simulink model "gm_sampleModel1995_3_sub_sub"  (R2023a)
settings: Solver=VariableStepAuto  StartTime=0.0  StopTime=10.0  RelTol=1e-3
libraries: hdlsllib x3, simulink x1
settings Model: Creator=user1  LastModifiedBy=user1
settings OptimizationCC: BlockReduction=off  ConditionallyExecuteInputs=off
settings DebuggingCC: InheritedTsInSrcMsg=none

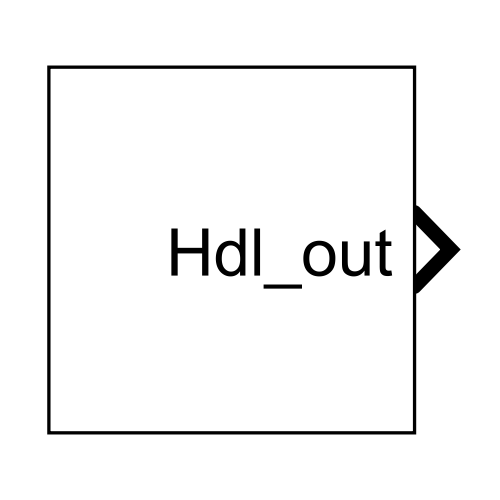
[thumbnail: Simulink's stored preview of the top-level diagram]
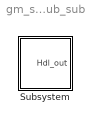
== system gm_sampleModel1995_3_sub_sub ==
  Subsystem : Subsystem

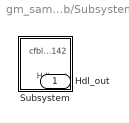
== system gm_sampleModel1995_3_sub_sub/Subsystem ==
  Subsystem : Subsystem
  Hdl_out : Outport  OutDataTypeStr=uint8

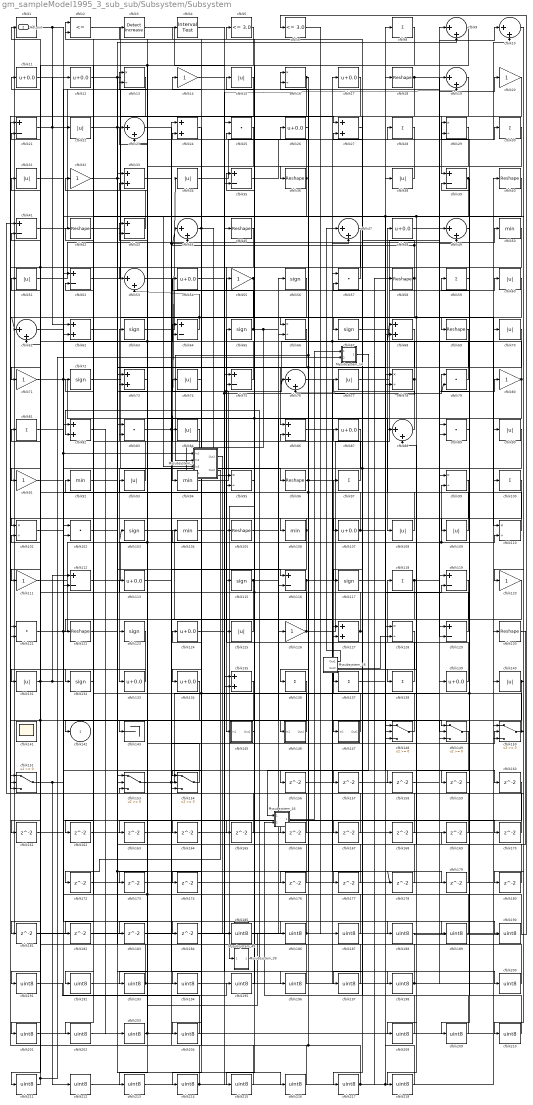
== system gm_sampleModel1995_3_sub_sub/Subsystem/Subsystem ==
  Mysubsystem_14 : Subsystem  TreatAsAtomicUnit=on  RTWFcnName=Mysubsystem_14
      settings: RTWFcnNameOpts=User specified  RTWFileNameOpts=Use function name
  Mysubsystem_16 : Subsystem  TreatAsAtomicUnit=on  RTWFcnName=Mysubsystem_16
      settings: RTWFcnNameOpts=User specified  RTWFileNameOpts=Use function name
  Mysubsystem_39 : Subsystem  TreatAsAtomicUnit=on  RTWFcnName=Mysubsystem_39
      settings: RTWFcnNameOpts=User specified  RTWFileNameOpts=Use function name
  Mysubsystem_44 : Subsystem  TreatAsAtomicUnit=on  RTWFcnName=Mysubsystem_44
      settings: RTWFcnNameOpts=User specified  RTWFileNameOpts=Use function name
  Mysubsystem_49 : Subsystem  TreatAsAtomicUnit=on  RTWFcnName=Mysubsystem_49
      settings: RTWFcnNameOpts=User specified  RTWFileNameOpts=Use function name
  Mysubsystem_7 : Subsystem  TreatAsAtomicUnit=on  RTWFcnName=Mysubsystem_7
      settings: RTWFcnNameOpts=User specified  RTWFileNameOpts=Use function name
  cfblk1 : ArithShift  BitShiftNumber=8
  cfblk{9..10,19,23,44,47,49,53,61,76,88} (11 alike) : Sum  Inputs=|++  OutDataTypeStr=uint8
  cfblk{8,28,30,59,81,97,100,118,136..138} (11 alike) : Sum  Inputs=+  OutDataTypeStr=uint8
  cfblk{13,16,29,66,78,95,99,101,110,128} (10 alike) : Product  Inputs=*/  OutDataTypeStr=uint8  RndMeth=Zero  SaturateOnIntegerOverflow=on
  cfblk{25,57,79,83,89,102,121} (7 alike) : DotProduct  OutDataTypeStr=uint8
  cfblk{56,63,65,67,72,103,115,117,123,132} (10 alike) : Signum
  cfblk{50,92,94,104,106} (5 alike) : MinMax  OutDataTypeStr=uint8
  cfblk{18,36,40,42,45,58,69,96,105,122,130} (11 alike) : Reshape
  cfblk{11..12,17,26,48,54,87,107,113,124,133..134,139} (13 alike) : Bias  Bias=0.0  SaturateOnIntegerOverflow=off
  cfblk{15,22,31,34,38,51,60,70,74,77,84,90,93,108..109,125,131,140} (18 alike) : Abs  OutDataTypeStr=uint8  SaturateOnIntegerOverflow=off
  cfblk{14,20,32,55,71,80,91,111,120,126} (10 alike) : Gain  OutDataTypeStr=uint8
  cfblk{21,35,39,41,43,52,64,75,112,116,119,129} (12 alike) : Sum  Inputs=+-  OutDataTypeStr=uint8
  cfblk{24,27,33,62,68,73,82,86,127,135} (10 alike) : Sum  OutDataTypeStr=uint8
  cfblk141 : Scope
      settings: Floating=on
  cfblk143 : Terminator
  cfblk145 : Subsystem
      settings: LibrarySourceBlock=|
      | hdlsllib/Ports &
      | Subsystems/Subsystem
  cfblk146 : Subsystem
      settings: LibrarySourceBlock=|
      | hdlsllib/Ports &
      | Subsystems/Subsystem
  cfblk147 : Subsystem
      settings: LibrarySourceBlock=|
      | hdlsllib/Ports &
      | Subsystems/Subsystem
  cfblk{148..151,153..154} (6 alike) : Switch  OutDataTypeStr=uint8  SaturateOnIntegerOverflow=off  InputSameDT=off
  cfblk{156..170,172..174,176..184} (27 alike) : Delay  SampleTime=1
  cfblk{185..198,200..204,208..218} (30 alike) : DataTypeConversion  OutDataTypeStr=uint8  SaturateOnIntegerOverflow=off  RndMeth=Floor
  cfblk2 : RelationalOperator  Operator=<=  OutDataTypeStr=boolean  InputSameDT=off
  cfblk3 : simulink/Logic and Bit Operations/Detect Increase  vinit=0.0  OutDataTypeStr=uint8
      settings: LibrarySourceBlock=|
      | hdlsllib/Logic and Bit
      | Operations/Detect
      | Increase
  cfblk4 : hdlsllib/Logic and Bit Operations/Interval Test  IntervalClosedRight=on  uplimit=0.5  IntervalClosedLeft=on  lowlimit=-0.5  OutDataTypeStr=uint8
  cfblk5 : hdlsllib/Logic and Bit Operations/Compare To Constant  relop=<=  const=3.0  OutDataTypeStr=uint8
  cfblk6 : hdlsllib/Logic and Bit Operations/Compare To Constant  relop=<=  const=3.0  OutDataTypeStr=uint8
  cfblk142 : Outport  OutDataTypeStr=uint8  VectorParamsAs1DForOutWhenUnconnected=off
  Hdl_out : Outport  Port=2  OutDataTypeStr=uint8
  wires:
  cfblk50/1 -> cfblk145/1(In1)
  cfblk84/1 -> cfblk133/1
  cfblk2/1 -> cfblk120/1
  cfblk69/1 -> cfblk156/1, cfblk153/2
  cfblk1/1 -> cfblk190/1, cfblk62/1
  cfblk20/1 -> cfblk39/1
  cfblk53/1 -> cfblk94/1
  cfblk139/1 -> cfblk65/1
  cfblk55/1 -> cfblk202/1, cfblk5/1
  cfblk64/1 -> cfblk53/2, cfblk61/1
  cfblk38/1 -> cfblk36/1
  cfblk83/1 -> cfblk115/1, cfblk34/1
  cfblk151/1 -> cfblk212/1, cfblk16/2
  cfblk48/1 -> cfblk49/1
  cfblk109/1 -> cfblk48/1
  cfblk56/1 -> cfblk111/1
  cfblk77/1 -> cfblk60/1
  cfblk65/1 -> cfblk54/1, cfblk67/1, Mysubsystem_7/4(In4)
  cfblk110/1 -> cfblk79/1
  cfblk138/1 -> cfblk118/1
  cfblk45/1 -> cfblk121/2, cfblk71/1
  cfblk32/1 -> cfblk96/1, cfblk216/1, cfblk178/1
  cfblk126/1 -> cfblk74/1, cfblk20/1
  cfblk67/1 -> cfblk10/1
  cfblk128/1 -> cfblk217/1
  cfblk6/1 -> cfblk187/1
  cfblk68/1 -> cfblk86/1
  cfblk135/1 -> cfblk211/1
  cfblk147/1(Out1) -> cfblk97/1
  cfblk63/1 -> cfblk38/1
  cfblk60/1 -> cfblk164/1, cfblk138/1
  cfblk121/1 -> cfblk95/2, cfblk17/1
  cfblk74/1 -> cfblk134/1
  cfblk97/1 -> cfblk63/1
  cfblk133/1 -> cfblk131/1
  cfblk16/1 -> cfblk161/1, cfblk146/1(In1)
  cfblk146/1(Out1) -> cfblk83/2, cfblk103/1
  cfblk153/1 -> cfblk150/2, cfblk89/1
  cfblk99/1 -> cfblk132/1
  cfblk24/1 -> cfblk214/1
  cfblk66/1 -> cfblk105/1
  cfblk70/1 -> cfblk147/1(In1)
  cfblk28/1 -> cfblk154/1
  cfblk82/1 -> cfblk203/1
  cfblk127/1 -> cfblk64/2, cfblk77/1
  cfblk88/1 -> cfblk57/2
  cfblk41/1 -> cfblk13/1
  cfblk103/1 -> cfblk125/1
  cfblk19/1 -> cfblk61/2
  cfblk42/1 -> cfblk129/2
  cfblk47/1 -> cfblk102/2
  cfblk112/1 -> cfblk19/1
  cfblk30/1 -> cfblk66/1
  cfblk22/1 -> cfblk78/2, cfblk27/1
  cfblk11/1 -> cfblk149/2, Mysubsystem_7/1(In1)
  cfblk15/1 -> cfblk91/1
  cfblk12/1 -> cfblk200/1, cfblk110/1
  cfblk58/1 -> cfblk117/1, cfblk3/1, cfblk44/1
  cfblk108/1 -> cfblk42/1
  cfblk154/1 -> cfblk93/1
  cfblk36/1 -> cfblk2/1, Mysubsystem_7/3(In3)
  cfblk52/1 -> cfblk9/1
  cfblk34/1 -> cfblk10/2
  cfblk18/1 -> cfblk107/1, cfblk89/2
  cfblk150/1 -> cfblk180/1, cfblk29/2, cfblk52/2, cfblk84/1
  cfblk72/1 -> cfblk108/1
  cfblk107/1 -> cfblk110/2, cfblk81/1, cfblk16/1
  cfblk3/1 -> cfblk75/1
  cfblk111/1 -> cfblk70/1, cfblk99/2
  cfblk105/1 -> cfblk56/1
  cfblk117/1 -> cfblk119/2
  cfblk134/1 -> cfblk181/1, cfblk151/2
  cfblk40/1 -> cfblk148/2, cfblk142/1
  cfblk122/1 -> cfblk73/1
  cfblk73/1 -> cfblk143/1
  cfblk51/1 -> cfblk50/1
  cfblk94/1 -> cfblk40/1
  cfblk71/1 -> cfblk64/1, cfblk126/1
  cfblk118/1 -> cfblk173/1, cfblk80/1
  cfblk93/1 -> cfblk2/2
  cfblk35/1 -> cfblk30/1
  cfblk25/1 -> cfblk193/1
  cfblk49/1 -> cfblk29/1
  cfblk140/1 -> cfblk177/1, cfblk41/1
  cfblk96/1 -> cfblk159/1, cfblk136/1
  cfblk116/1 -> cfblk154/3, cfblk28/1, cfblk68/1
  cfblk80/1 -> cfblk51/1, cfblk215/1, cfblk123/1
  cfblk78/1 -> cfblk76/2, cfblk43/1
  cfblk131/1 -> cfblk41/2, cfblk112/1, cfblk22/1
  cfblk5/1 -> cfblk183/1, cfblk182/1
  cfblk21/1 -> cfblk12/1, cfblk49/2
  cfblk57/1 -> cfblk35/1
  cfblk43/1 -> cfblk32/1
  cfblk13/1 -> cfblk151/3
  cfblk86/1 -> cfblk88/1
  cfblk125/1 -> cfblk122/1
  cfblk79/1 -> cfblk27/2
  cfblk145/1(Out1) -> cfblk15/1
  cfblk33/1 -> cfblk44/2, cfblk127/2
  cfblk90/1 -> cfblk112/2, cfblk137/1
  cfblk89/1 -> cfblk109/1
  cfblk106/1 -> cfblk154/2, cfblk101/1
  cfblk75/1 -> cfblk21/2, cfblk33/2
  cfblk115/1 -> cfblk163/1, cfblk149/1
  cfblk92/1 -> cfblk76/1, cfblk75/2
  cfblk44/1 -> cfblk174/1, cfblk95/1
  cfblk39/1 -> cfblk69/1, cfblk208/1, cfblk148/3
  cfblk124/1 -> cfblk19/2, cfblk79/2
  cfblk132/1 -> cfblk72/1
  cfblk148/1 -> cfblk124/1
  cfblk29/1 -> cfblk53/1
  cfblk102/1 -> cfblk9/2
  cfblk129/1 -> cfblk11/1, cfblk55/1
  cfblk17/1 -> cfblk106/1, Mysubsystem_7/2(In2)
  cfblk62/1 -> cfblk116/1
  cfblk23/1 -> cfblk198/1
  cfblk156/1 -> cfblk129/1
  cfblk27/1 -> cfblk157/1
  cfblk157/1 -> cfblk148/1
  cfblk61/1 -> cfblk158/1
  cfblk158/1 -> cfblk99/1
  cfblk159/1 -> cfblk39/2
  cfblk137/1 -> cfblk160/1
  cfblk161/1 -> cfblk62/2
  cfblk87/1 -> cfblk162/1
  cfblk162/1 -> cfblk150/1
  cfblk163/1 -> cfblk78/1
  cfblk164/1 -> cfblk119/1
  cfblk9/1 -> cfblk165/1
  cfblk165/1 -> cfblk151/1
  cfblk101/1 -> cfblk166/1
  cfblk166/1 -> cfblk43/2
  cfblk113/1 -> cfblk167/1
  cfblk167/1 -> cfblk83/1
  cfblk168/1 -> cfblk127/1
  cfblk130/1 -> cfblk169/1
  cfblk169/1 -> cfblk1/1
  cfblk54/1 -> cfblk170/1
  cfblk170/1 -> cfblk13/2
  cfblk172/1 -> cfblk149/3
  cfblk173/1 -> cfblk150/3
  cfblk174/1 -> cfblk66/2
  cfblk26/1 -> cfblk176/1
  cfblk176/1 -> cfblk153/1
  cfblk177/1 -> cfblk153/3
  cfblk178/1 -> cfblk86/2
  cfblk76/1 -> cfblk179/1
  cfblk179/1 -> cfblk57/1
  cfblk180/1 -> cfblk88/2
  cfblk181/1 -> cfblk35/2
  cfblk182/1 -> cfblk68/2
  cfblk183/1 -> cfblk116/2
  cfblk81/1 -> cfblk184/1
  cfblk184/1 -> cfblk18/1
  cfblk4/1 -> cfblk185/1
  cfblk185/1 -> cfblk90/1
  cfblk31/1 -> cfblk186/1
  cfblk186/1 -> Hdl_out/1, cfblk4/1
  cfblk187/1 -> cfblk102/1, cfblk113/1
  cfblk91/1 -> cfblk188/1
  cfblk188/1 -> cfblk6/1
  cfblk104/1 -> cfblk189/1
  cfblk189/1 -> cfblk92/1
  cfblk190/1 -> cfblk104/1
  cfblk100/1 -> cfblk191/1
  cfblk123/1 -> cfblk192/1
  cfblk192/1 -> cfblk100/1
  cfblk193/1 -> cfblk47/2, cfblk101/2
  cfblk120/1 -> cfblk194/1
  cfblk194/1 -> cfblk25/1
  cfblk191/1 -> cfblk195/1
  cfblk195/1 -> cfblk25/2
  cfblk14/1 -> cfblk196/1
  cfblk196/1 -> cfblk33/1
  cfblk119/1 -> cfblk197/1
  cfblk197/1 -> cfblk14/1
  cfblk198/1 -> cfblk52/1, cfblk139/1
  cfblk200/1 -> cfblk23/2
  cfblk8/1 -> cfblk201/1
  cfblk201/1 -> cfblk45/1
  cfblk202/1 -> cfblk8/1
  cfblk203/1 -> cfblk140/1, cfblk73/2
  cfblk136/1 -> cfblk204/1
  cfblk204/1 -> cfblk82/1
  cfblk59/1 -> cfblk209/1
  cfblk209/1 -> cfblk87/1
  cfblk10/1 -> cfblk210/1
  cfblk210/1 -> cfblk59/1
  cfblk211/1 -> cfblk31/1, Mysubsystem_14/2(In2)
  cfblk212/1 -> cfblk135/1
  cfblk160/1 -> cfblk213/1
  cfblk213/1 -> cfblk135/2
  cfblk214/1 -> cfblk21/1, cfblk130/1, cfblk168/1
  cfblk215/1 -> cfblk24/1
  cfblk216/1 -> cfblk24/2
  cfblk217/1 -> cfblk58/1, cfblk26/1, cfblk121/1
  cfblk149/1 -> cfblk218/1
  cfblk218/1 -> cfblk128/1
  Mysubsystem_7/2(Out2) -> cfblk172/1
  Mysubsystem_16/1(Out1) -> cfblk47/1
  Mysubsystem_16/2(Out2) -> cfblk128/2
  cfblk95/1 -> Mysubsystem_39/1(In1)
  Mysubsystem_39/1(Out1) -> cfblk82/2
  Mysubsystem_14/1(Out1) -> Mysubsystem_44/1(In1)
  cfblk208/1 -> Mysubsystem_44/2(In2)
  Mysubsystem_44/1(Out1) -> Mysubsystem_14/1(In1)
  Mysubsystem_7/1(Out1) -> Mysubsystem_49/1(In1)
  Mysubsystem_49/1(Out1) -> cfblk23/1

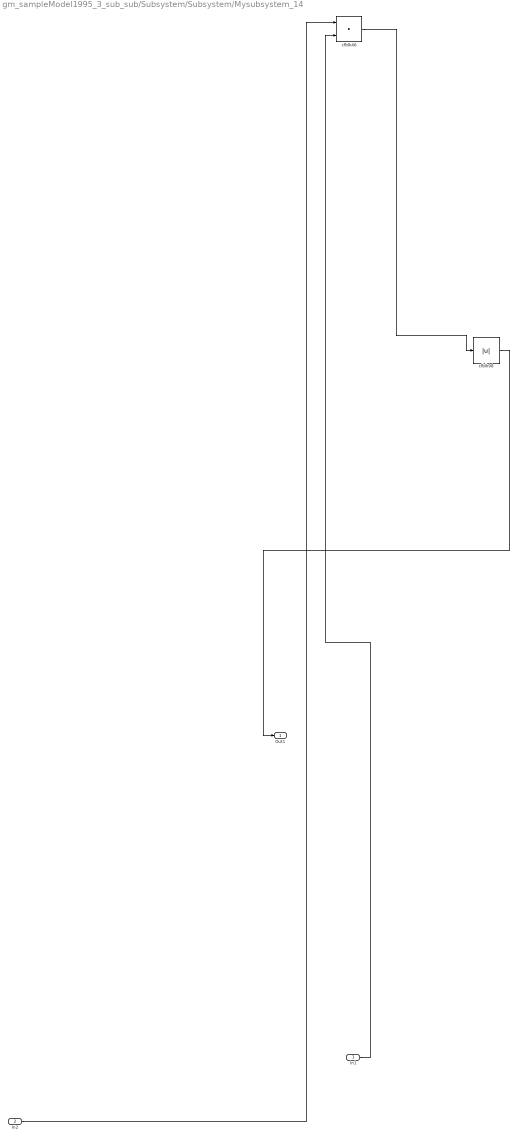
== system gm_sampleModel1995_3_sub_sub/Subsystem/Subsystem/Mysubsystem_14 ==
  In1 : Inport
  In2 : Inport  Port=2
  cfblk46 : DotProduct  OutDataTypeStr=Inherit: Inherit via internal rule
  cfblk98 : Abs  SaturateOnIntegerOverflow=off
  Out1 : Outport
  wires:
  In1/1 -> cfblk46/2
  In2/1 -> cfblk46/1
  cfblk98/1 -> Out1/1
  cfblk46/1 -> cfblk98/1

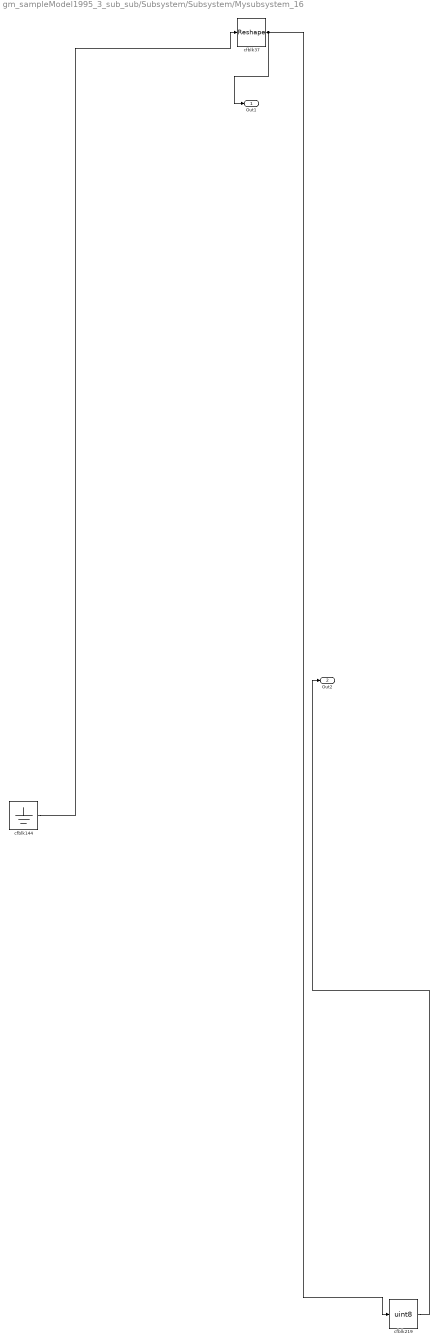
== system gm_sampleModel1995_3_sub_sub/Subsystem/Subsystem/Mysubsystem_16 ==
  cfblk144 : Ground
  cfblk219 : DataTypeConversion  OutDataTypeStr=uint8  SaturateOnIntegerOverflow=off  RndMeth=Floor
  cfblk37 : Reshape
  Out1 : Outport
  Out2 : Outport  Port=2
  wires:
  cfblk219/1 -> Out2/1
  cfblk144/1 -> cfblk37/1
  cfblk37/1 -> cfblk219/1, Out1/1

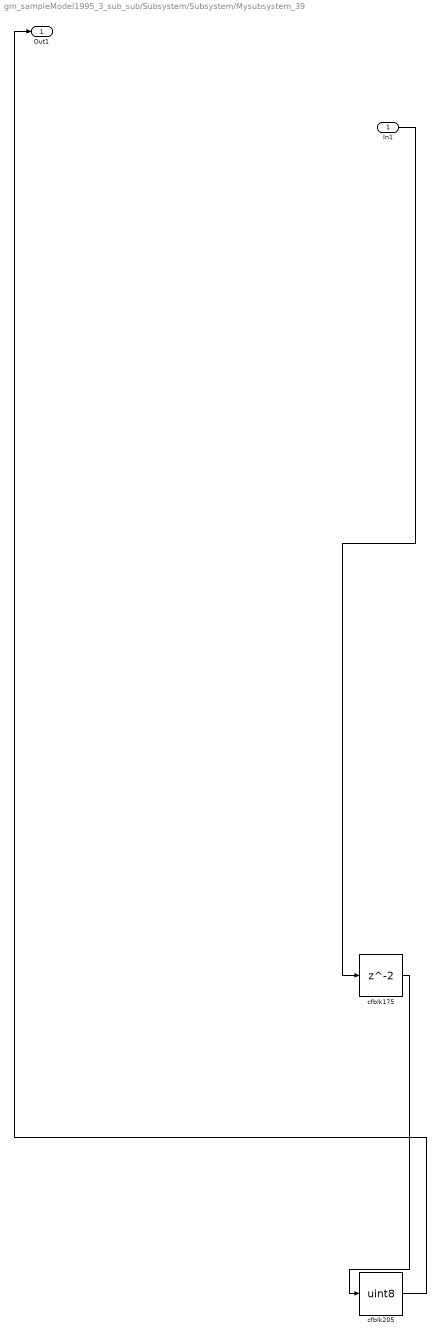
== system gm_sampleModel1995_3_sub_sub/Subsystem/Subsystem/Mysubsystem_39 ==
  In1 : Inport
  cfblk175 : Delay  SampleTime=1
  cfblk205 : DataTypeConversion  OutDataTypeStr=uint8  SaturateOnIntegerOverflow=off  RndMeth=Floor
  Out1 : Outport
  wires:
  cfblk205/1 -> Out1/1
  In1/1 -> cfblk175/1
  cfblk175/1 -> cfblk205/1

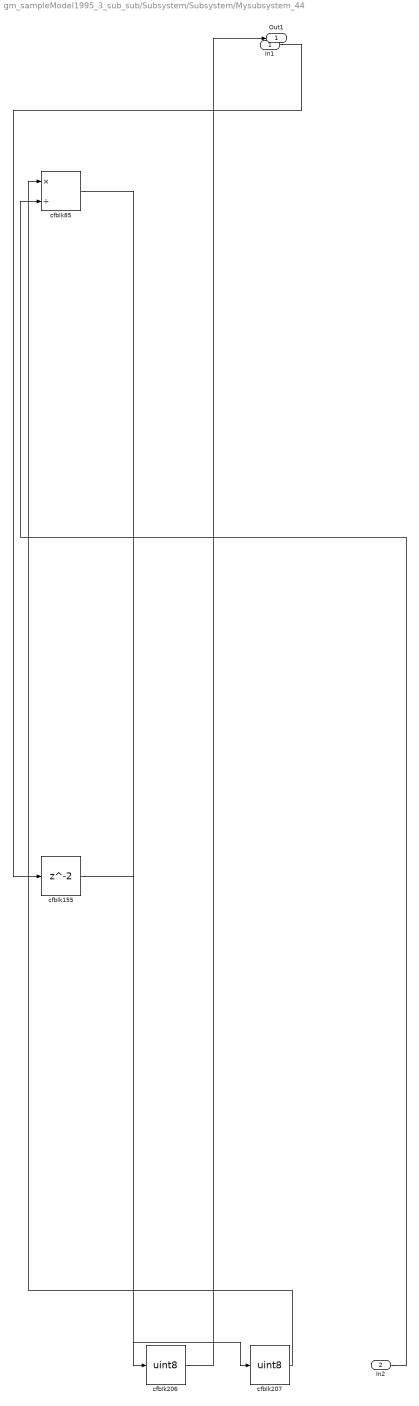
== system gm_sampleModel1995_3_sub_sub/Subsystem/Subsystem/Mysubsystem_44 ==
  In1 : Inport
  In2 : Inport  Port=2
  cfblk155 : Delay  SampleTime=1
  cfblk206 : DataTypeConversion  OutDataTypeStr=uint8  SaturateOnIntegerOverflow=off  RndMeth=Floor
  cfblk207 : DataTypeConversion  OutDataTypeStr=uint8  SaturateOnIntegerOverflow=off  RndMeth=Floor
  cfblk85 : Product  Inputs=*/  RndMeth=Zero  SaturateOnIntegerOverflow=on
  Out1 : Outport
  wires:
  cfblk206/1 -> Out1/1
  In1/1 -> cfblk155/1
  cfblk155/1 -> cfblk207/1
  In2/1 -> cfblk85/2
  cfblk85/1 -> cfblk206/1
  cfblk207/1 -> cfblk85/1

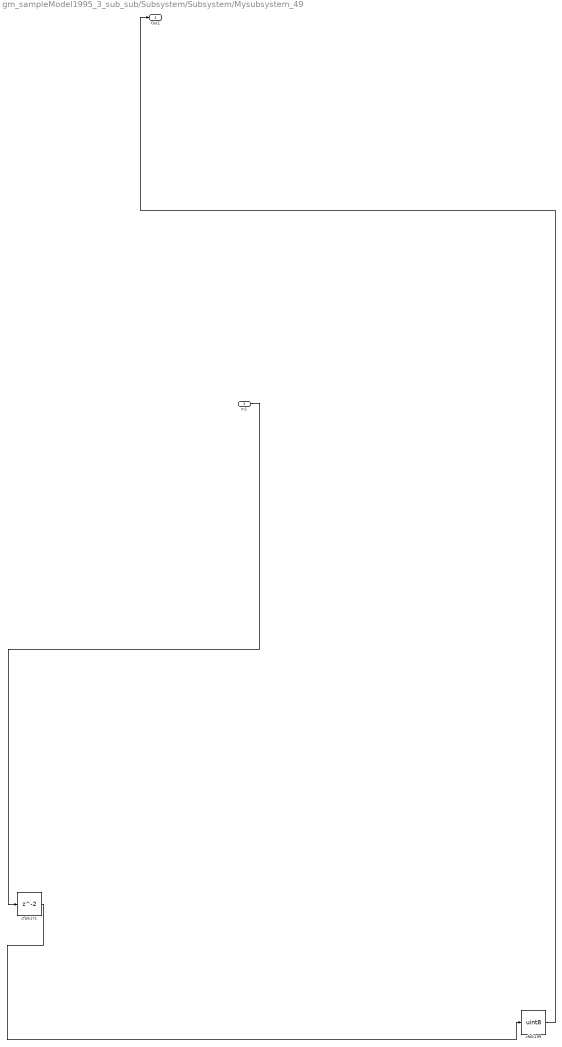
== system gm_sampleModel1995_3_sub_sub/Subsystem/Subsystem/Mysubsystem_49 ==
  In1 : Inport
  cfblk171 : Delay  SampleTime=1
  cfblk199 : DataTypeConversion  OutDataTypeStr=uint8  SaturateOnIntegerOverflow=off  RndMeth=Floor
  Out1 : Outport
  wires:
  cfblk199/1 -> Out1/1
  In1/1 -> cfblk171/1
  cfblk171/1 -> cfblk199/1

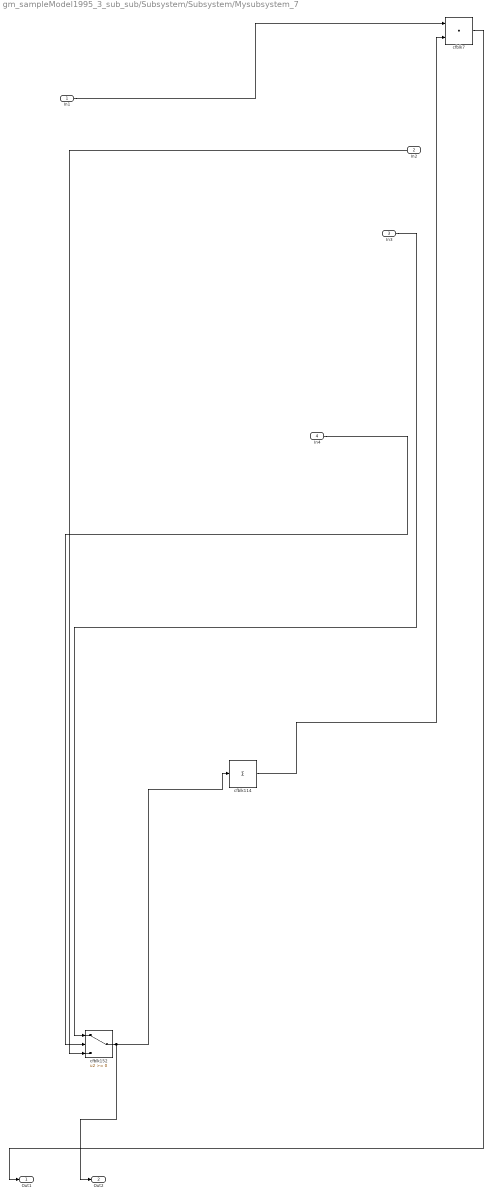
== system gm_sampleModel1995_3_sub_sub/Subsystem/Subsystem/Mysubsystem_7 ==
  In1 : Inport
  In2 : Inport  Port=2
  In3 : Inport  Port=3
  In4 : Inport  Port=4
  cfblk114 : Sum  Inputs=+
  cfblk152 : Switch  SaturateOnIntegerOverflow=off  InputSameDT=off
  cfblk7 : DotProduct  OutDataTypeStr=Inherit: Inherit via internal rule
  Out1 : Outport
  Out2 : Outport  Port=2
  wires:
  In1/1 -> cfblk7/1
  In3/1 -> cfblk152/1
  In2/1 -> cfblk152/3
  In4/1 -> cfblk152/2
  cfblk7/1 -> Out1/1
  cfblk114/1 -> cfblk7/2
  cfblk152/1 -> cfblk114/1, Out2/1

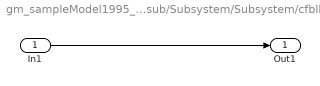
== system gm_sampleModel1995_3_sub_sub/Subsystem/Subsystem/cfblk145 ==
  In1 : Inport
  Out1 : Outport
  wires:
  In1/1 -> Out1/1

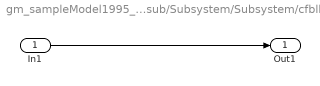
== system gm_sampleModel1995_3_sub_sub/Subsystem/Subsystem/cfblk146 ==
  In1 : Inport
  Out1 : Outport
  wires:
  In1/1 -> Out1/1

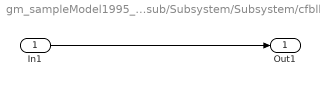
== system gm_sampleModel1995_3_sub_sub/Subsystem/Subsystem/cfblk147 ==
  In1 : Inport
  Out1 : Outport
  wires:
  In1/1 -> Out1/1
